simulink model "massforce"  (R2018b)
settings: Solver=VariableStepAuto  StartTime=0.0  StopTime=10.0  RelTol=1e-3
settings Model: Creator=prakyath  LastModifiedBy=prakyath
settings DebuggingCC: LibraryContextMissingDiagnostic=none
settings SFSimCC: SimUseLocalCustomCode=off
settings RTWCC: RTWUseLocalCustomCode=off

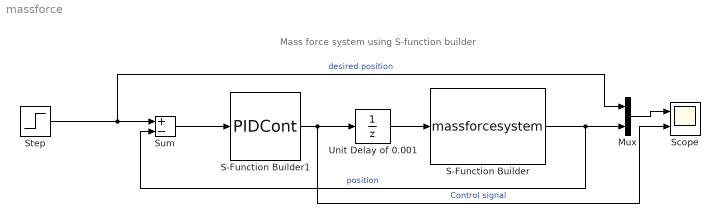
== system massforce ==
  note: Mass force system using S-function builder
  Mux : Mux  Inputs=2
  "S-Function Builder " : S-Function  InitFcn=try, set_param(gcb,'FunctionName','massforcesystem'), end  FunctionName=massforcesystem  Parameters=0,5,1,0.001  SFunctionModules=massforcesystem_wrapper massc  SFunctionDeploymentMode=off  EnableBusSupport=off  mask(S-Function Builder){}
      mask help: Simulink:masks:SFunctionBuilder_MD
      mask init:
      | val = [[.9  0.75 0.75 1 1 .9 .9 1]',[1 1 0.75 0.75 .9 .9 1 .9]'];try , sys = get_param(gcb,'SfunBuilderFcnName');if isempty(sys), sys = get_param(gcb,'FunctionName'); end,catch, sys = get_param(gcb,'FunctionName'); end
      settings: CopyFcn=set_param(gcbh,'LinkStatus','none')  PreSaveFcn=try, set_param(gcb,'FunctionName','massforcesystem'), end  OpenFcn=sfunctionwizard(gcbh)
      mask Display:
      | plot(val(:,1),val(:,2))
      | disp(sys)
      | port_label('input',1,'u1')
      | port_label('output',1,'y1')
  "S-Function Builder1 " : S-Function  InitFcn=try, set_param(gcb,'FunctionName','PIDCont'), end  FunctionName=PIDCont  Parameters=25,0,5  SFunctionModules=PIDCont_wrapper PIDC  SFunctionDeploymentMode=off  EnableBusSupport=off  mask(S-Function Builder){}
      mask help: Simulink:masks:SFunctionBuilder_MD
      mask init: same as massforce/S-Function Builder 
      settings: CopyFcn=set_param(gcbh,'LinkStatus','none')  PreSaveFcn=try, set_param(gcb,'FunctionName','PIDCont'), end  OpenFcn=sfunctionwizard(gcbh)
      mask Display: plot(val(:,1),val(:,2)),disp(sys), port_label('input',1,'u0'), port_label('output',1,'y0')
  Scope : Scope  NumInputPorts=2
  Step : Step  SampleTime=0
  Sum : Sum  Inputs=+-
  Unit Delay of 0.001 : UnitDelay  SampleTime=0.001
  wires:
  Step/1 -> Mux/1, Sum/1  "desired position"
  "S-Function Builder "/1 -> Sum/2, Mux/2  "position"
  "S-Function Builder1 "/1 -> Scope/2, Unit Delay of 0.001/1  "Control signal"
  Sum/1 -> "S-Function Builder1 "/1
  Unit Delay of 0.001/1 -> "S-Function Builder "/1
  Mux/1 -> Scope/1
